simulink model "Thrust"  (R2015a)
settings: Solver=ode45  StartTime=0.0  StopTime=22.86  RelTol=1e-3
settings Model: Creator=Nick  LastModifiedBy=Nick

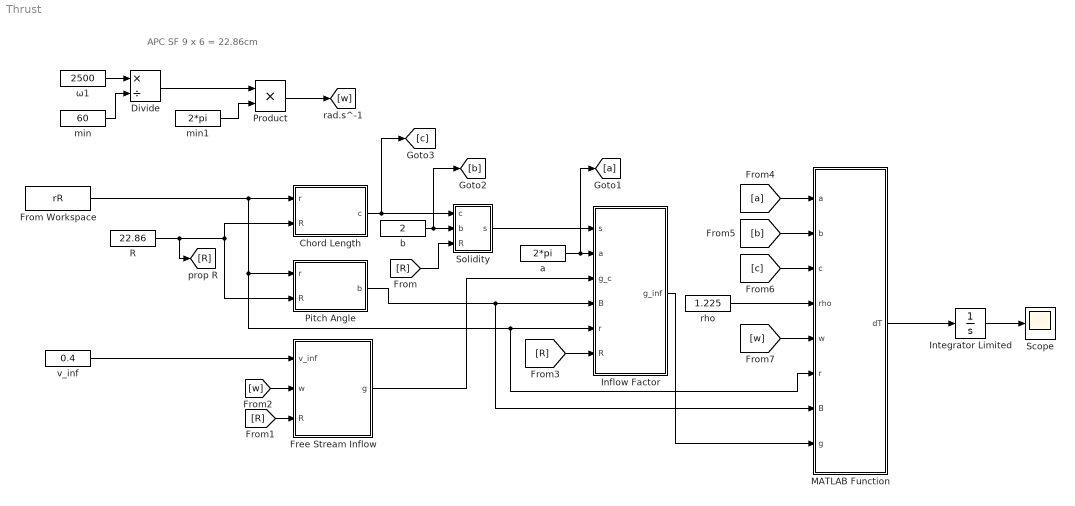
== system Thrust ==
  note: APC SF 9 x 6 = 22.86cm
  Chord Length : MATLAB Function  TreatAsAtomicUnit=on
  Divide : Product  Inputs=*/
  Free Stream Inflow : MATLAB Function  TreatAsAtomicUnit=on
  From Workspace : FromWorkspace  VariableName=rR  SampleTime=0  OutputAfterFinalValue=Holding final value
  Inflow Factor : MATLAB Function  TreatAsAtomicUnit=on
  Integrator Limited : Integrator  UpperSaturationLimit=1  LowerSaturationLimit=0
  MATLAB Function : MATLAB Function  TreatAsAtomicUnit=on
  Pitch Angle : MATLAB Function  TreatAsAtomicUnit=on
  Product : Product
  R : Constant  Value=22.86
  Scope : Scope
  Solidity : MATLAB Function  TreatAsAtomicUnit=on
  a : Constant  Value=2*pi
  b : Constant  Value=2
  min : Constant  Value=60
  min1 : Constant  Value=2*pi
  rho : Constant  Value=1.225
  v_inf : Constant  Value=0.4
  ω1 : Constant  Value=2500
  wires:
  R/1 -> [R], Pitch Angle/2(R), Chord Length/2(R)
  From Workspace/1 -> MATLAB Function/6(r), Inflow Factor/5(r), Pitch Angle/1(r), Chord Length/1(r)
  Chord Length/1(c) -> [c], Solidity/1(c)
  Pitch Angle/1(b) -> MATLAB Function/7(B), Inflow Factor/4(B)
  [R] -> Solidity/3(R)
  [R] -> Free Stream Inflow/3(R)
  [w] -> Free Stream Inflow/2(w)
  v_inf/1 -> Free Stream Inflow/1(v_inf)
  Solidity/1(s) -> Inflow Factor/1(s)
  a/1 -> [a], Inflow Factor/2(a)
  Free Stream Inflow/1(g) -> Inflow Factor/3(g_c)
  [R] -> Inflow Factor/6(R)
  ω1/1 -> Divide/1
  min/1 -> Divide/2
  Divide/1 -> Product/1
  min1/1 -> Product/2
  Product/1 -> [w]
  [a] -> MATLAB Function/1(a)
  b/1 -> [b], Solidity/2(b)
  [b] -> MATLAB Function/2(b)
  [c] -> MATLAB Function/3(c)
  rho/1 -> MATLAB Function/4(rho)
  [w] -> MATLAB Function/5(w)
  Inflow Factor/1(g_inf) -> MATLAB Function/8(g)
  Integrator Limited/1 -> Scope/1
  MATLAB Function/1(dT) -> Integrator Limited/1

== matlab function Thrust/Pitch Angle ==
  data: r input; b output; R input
function b = Br(r,R)
x = r/R;
%pitch angle (rad)
b = - (731*x^6)/20 + 138*x^5 - 210*x^4 + (1637*x^3)/10 - (3383*x^2)/50 + (643*x)/50 - 2003/10000;
end

== matlab function Thrust/Chord Length ==
  data: r input; c output; R input
function c = Cr(r,R)
x = r/R;
%Chord Length (m^-3)
y = (5623*x^6)/1000 - (2221*x^5)/100 + (173*x^4)/5 - (683*x^3)/25 + (1079*x^2)/100 - (813*x)/500 + 1987/10000;
c = y*10^-3;
end

== matlab function Thrust/Solidity ==
  data: c input; b input; s output; R input
function s = sigma(c,b,R)
s = (b*c)/(pi*R);
end

== matlab function Thrust/Free Stream Inflow ==
  data: v_inf input; g output; w input; R input
function g = gamma_c(v_inf,w,R)
%#codegen
g=(v_inf)/(w*(R*10^-3));
end

== matlab function Thrust/Inflow Factor ==
  data: s input; g_inf output; a input; g_c input; B input; r input; R input
function g_inf = gamma(s,a,g_c,B,r,R)
g_inf = sqrt((s*a/16 - g_c/2)^2 + (s*a/8)*B*(r/R))-(s*a/16 - g_c/2);
end

== matlab function Thrust/MATLAB Function ==
  data: a input; dT output; b input; c input; rho input; w input; r input; B input; g input
function dT = thrust(a,b,c,rho,w,r,B,g)
dT = a*b*c*(1/2)*rho*((w*r)^2)*(B-g);
end
